simulink model "double_track_dynamics_model"  (R2023b)
settings: Solver=VariableStepAuto  StartTime=0.0  StopTime=10.0  RelTol=1e-3
undefined symbols (not defined in the file or in its folder): a, b, mass_total, track_width_front, track_width_rear, yaw_polar_inertia
settings Model: Creator=bglen  LastModifiedBy=bglen

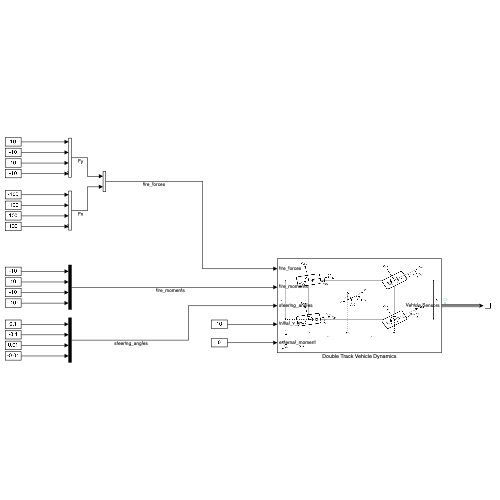
[thumbnail: Simulink's stored preview of the top-level diagram]
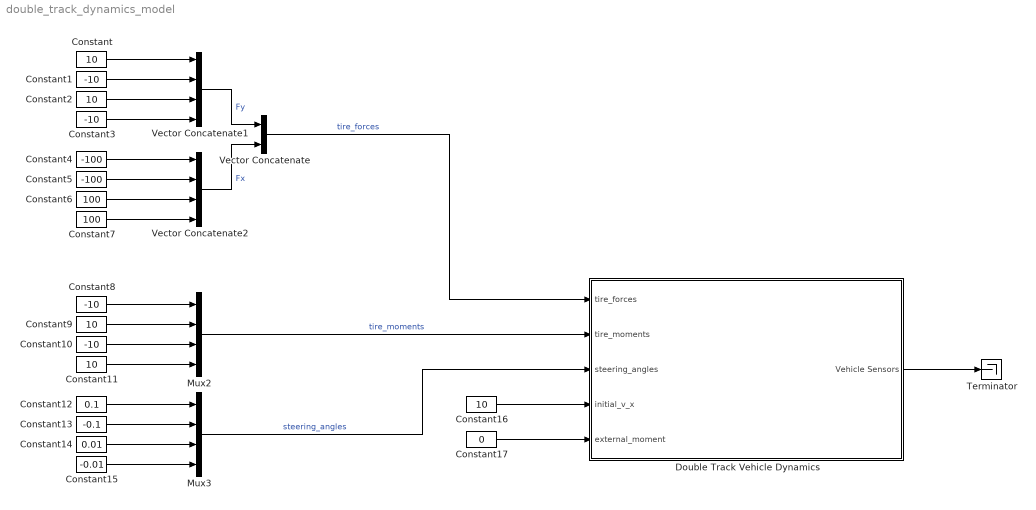
== system double_track_dynamics_model ==
  Constant{,2,9,11,16} (5 alike) : Constant  Value=10
  Constant{1,3,8,10} (4 alike) : Constant  Value=-10
  Constant12 : Constant  Value=0.1
  Constant13 : Constant  Value=-0.1
  Constant14 : Constant  Value=0.01
  Constant15 : Constant  Value=-0.01
  Constant17 : Constant  Value=0
  Constant4 : Constant  Value=-100
  Constant5 : Constant  Value=-100
  Constant6 : Constant  Value=100
  Constant7 : Constant  Value=100
  Double Track Vehicle Dynamics : Subsystem
      mask Display: image('double_track_diagram.png');
  Mux2 : Mux
  Mux3 : Mux
  Terminator : Terminator
  Vector Concatenate : Concatenate  Mode=Multidimensional array
  Vector Concatenate1 : Concatenate  NumInputs=4  Mode=Multidimensional array  ConcatenateDimension=2
  Vector Concatenate2 : Concatenate  NumInputs=4  Mode=Multidimensional array  ConcatenateDimension=2
  wires:
  Vector Concatenate/1 -> Double Track Vehicle Dynamics/1(tire_forces)  "tire_forces"
  Mux2/1 -> Double Track Vehicle Dynamics/2(tire_moments)  "tire_moments"
  Mux3/1 -> Double Track Vehicle Dynamics/3(steering_angles)  "steering_angles"
  Constant16/1 -> Double Track Vehicle Dynamics/4(initial_v_x)
  Double Track Vehicle Dynamics/1(Vehicle Sensors) -> Terminator/1
  Constant/1 -> Vector Concatenate1/1
  Constant2/1 -> Vector Concatenate1/3
  Constant3/1 -> Vector Concatenate1/4
  Constant6/1 -> Vector Concatenate2/3
  Constant7/1 -> Vector Concatenate2/4
  Constant4/1 -> Vector Concatenate2/1
  Constant5/1 -> Vector Concatenate2/2
  Vector Concatenate2/1 -> Vector Concatenate/2  "Fx"
  Constant9/1 -> Mux2/2
  Constant11/1 -> Mux2/4
  Constant8/1 -> Mux2/1
  Constant10/1 -> Mux2/3
  Constant13/1 -> Mux3/2
  Constant15/1 -> Mux3/4
  Constant12/1 -> Mux3/1
  Constant14/1 -> Mux3/3
  Constant1/1 -> Vector Concatenate1/2
  Vector Concatenate1/1 -> Vector Concatenate/1  "Fy"
  Constant17/1 -> Double Track Vehicle Dynamics/5(external_moment)

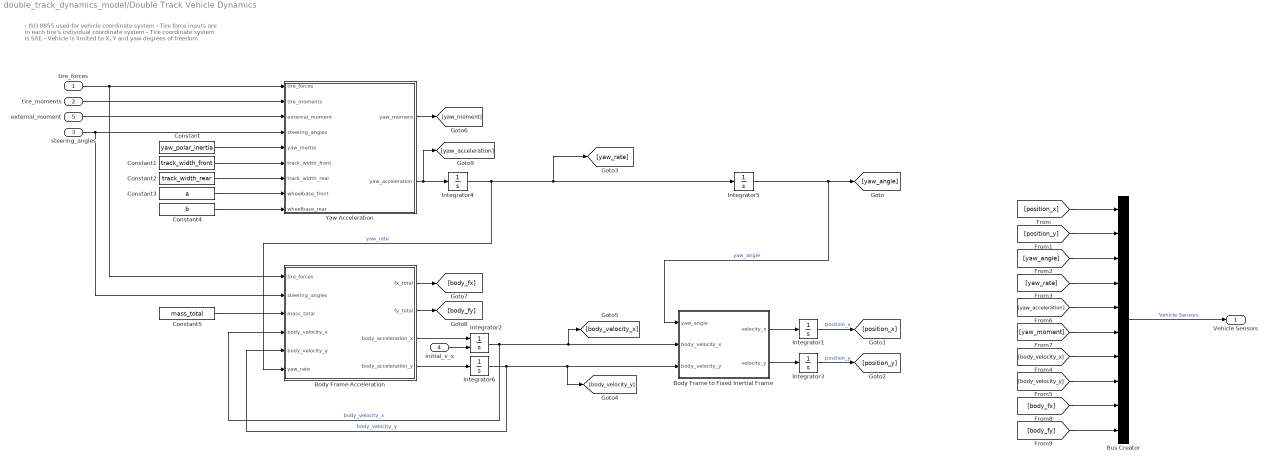
== system double_track_dynamics_model/Double Track Vehicle Dynamics ==
  note: - ISO 8855 used for vehicle coordinate system
      | - Tire force inputs are in each tire's individual coordinate system
      | - Tire coordinate system is SAE
      | - Vehicle is limited to X, Y and yaw degrees of freedom
  tire_forces : Inport
  tire_moments : Inport  Port=2
  steering_angles : Inport  Port=3
  initial_v_x : Inport  Port=4
  external_moment : Inport  Port=5
  Body Frame Acceleration : MATLAB Function  TreatAsAtomicUnit=on
  Body Frame to Fixed Inertial Frame : MATLAB Function  TreatAsAtomicUnit=on
  Bus Creator : BusCreator  Inputs=10
  Constant : Constant  Value=yaw_polar_inertia
  Constant1 : Constant  Value=track_width_front
  Constant2 : Constant  Value=track_width_rear
  Constant3 : Constant  Value=a
  Constant4 : Constant  Value=b
  Constant5 : Constant  Value=mass_total
  Integrator{1,3..6} (5 alike) : Integrator
  Integrator2 : Integrator  InitialConditionSource=external
  Yaw Acceleration : MATLAB Function  TreatAsAtomicUnit=on
  Vehicle Sensors : Outport
  wires:
  tire_moments/1 -> Yaw Acceleration/2(tire_moments)
  Bus Creator/1 -> Vehicle Sensors/1  "Vehicle Sensors"
  [yaw_rate] -> Bus Creator/4
  [position_y] -> Bus Creator/2
  Body Frame Acceleration/4(body_acceleration_y) -> Integrator6/1
  [position_x] -> Bus Creator/1
  steering_angles/1 -> Yaw Acceleration/4(steering_angles), Body Frame Acceleration/2(steering_angles)
  Integrator2/1 -> Body Frame Acceleration/4(body_velocity_x), [body_velocity_x], Body Frame to Fixed Inertial Frame/2(body_velocity_x)  "body_velocity_x"
  Body Frame to Fixed Inertial Frame/2(velocity_y) -> Integrator3/1
  Integrator1/1 -> [position_x]  "position_x"
  initial_v_x/1 -> Integrator2/2
  Integrator5/1 -> [yaw_angle], Body Frame to Fixed Inertial Frame/1(yaw_angle)  "yaw_angle"
  Integrator3/1 -> [position_y]  "position_y"
  [yaw_angle] -> Bus Creator/3
  Body Frame to Fixed Inertial Frame/1(velocity_x) -> Integrator1/1
  tire_forces/1 -> Body Frame Acceleration/1(tire_forces), Yaw Acceleration/1(tire_forces)
  Integrator4/1 -> Body Frame Acceleration/6(yaw_rate), [yaw_rate], Integrator5/1  "yaw_rate"
  Integrator6/1 -> Body Frame Acceleration/5(body_velocity_y), [body_velocity_y], Body Frame to Fixed Inertial Frame/3(body_velocity_y)  "body_velocity_y"
  Constant/1 -> Yaw Acceleration/5(yaw_inertia)
  Constant4/1 -> Yaw Acceleration/9(wheelbase_rear)
  Constant3/1 -> Yaw Acceleration/8(wheelbase_front)
  Constant2/1 -> Yaw Acceleration/7(track_width_rear)
  Constant1/1 -> Yaw Acceleration/6(track_width_front)
  Yaw Acceleration/2(yaw_acceleration) -> [yaw_acceleration], Integrator4/1
  Body Frame Acceleration/3(body_acceleration_x) -> Integrator2/1
  Constant5/1 -> Body Frame Acceleration/3(mass_total)
  Yaw Acceleration/1(yaw_moment) -> [yaw_moment]
  Body Frame Acceleration/1(fx_total) -> [body_fx]
  Body Frame Acceleration/2(fy_total) -> [body_fy]
  [yaw_acceleration] -> Bus Creator/5
  [yaw_moment] -> Bus Creator/6
  [body_velocity_x] -> Bus Creator/7
  [body_velocity_y] -> Bus Creator/8
  [body_fx] -> Bus Creator/9
  [body_fy] -> Bus Creator/10
  external_moment/1 -> Yaw Acceleration/3(external_moment)

== matlab function double_track_dynamics_model/Double Track Vehicle Dynamics/Body Frame Acceleration ==
  data: tire_forces input; steering_angles input; fx_total output; fy_total output; body_acceleration_x output; body_acceleration_y output; mass_total input; body_velocity_x input; body_velocity_y input; yaw_rate input
%{

Solve the equation of motion for longitudianl acceleration

Sum(Fx) / mass = long_acceleration

%% Inputs:

Tire Forces [N]: tire_forces = [fy_fl, fy_fr, fy_rl, fy_rr; fx_fl, fx_fr, fx_rl, fx_rr]; 
Steering Angles [rad]: steering_angles = [delta_fl, delta_fr, delta_rl, delta_rr];

%% Outputs:

fx_total [N]
fy_total [N]
body_acceleration_x [m/s^2]
body_acceleration_y [m/s^2]

%}
function [fx_total, fy_total, body_acceleration_x, body_acceleration_y]  = fcn(tire_forces, steering_angles, mass_total, body_velocity_x, body_velocity_y, yaw_rate)

%% convert input matricies into individual forces for code clarity
fy_fl = tire_forces(1, 1);
fy_fr = tire_forces(1, 2);
fy_rl = tire_forces(1, 3);
fy_rr = tire_forces(1, 4);

fx_fl = tire_forces(2, 1);
fx_fr = tire_forces(2, 2);
fx_rl = tire_forces(2, 3);
fx_rr = tire_forces(2, 4);

delta_fl = steering_angles(1);
delta_fr = steering_angles(2);
delta_rl = steering_angles(3);
delta_rr = steering_angles(4);

%% Convert tire forces into vehicle body frame
fx_body_fl = fy_fl * sin(delta_fl) + fx_fl * cos(delta_fl);
fy_body_fl = fy_fl * cos(delta_fl) + fx_fl * sin(delta_fl);

fx_body_fr = fy_fr * sin(delta_fr) + fx_fr * cos(delta_fr);
fy_body_fr = fy_fr * cos(delta_fr) + fx_fr * sin(delta_fr);

fx_body_rl = fy_rl * sin(delta_rl) + fx_rl * cos(delta_rl);
fy_body_rl = fy_rl * cos(delta_rl) + fx_rl * sin(delta_rl);

fx_body_rr = fy_rr * sin(delta_rr) + fx_rr * cos(delta_rr);
fy_body_rr = fy_rr * cos(delta_rr) + fx_rr * sin(delta_rr);

%% Calculate Longitudinal force and acceleration
fx_total = fx_body_fl + fx_body_fr + fx_body_rl + fx_body_rr;
body_acceleration_x = (fx_total / mass_total) - (yaw_rate * body_velocity_y); % must account for the apparent coriolis force

%% Calculate Lateral force and acceleration
fy_total = (fy_body_fl + fy_body_fr + fy_body_rl + fy_body_rr) + (yaw_rate * body_velocity_x); % must account for the apparent coriolis force
body_acceleration_y = fy_total / mass_total;

== matlab function double_track_dynamics_model/Double Track Vehicle Dynamics/Body Frame to Fixed Inertial Frame ==
  data: yaw_angle input; velocity_x output; body_velocity_x input; body_velocity_y input; velocity_y output
%{
%% Double Track Vehicle Dynamics

%% Overview
These equations describe the vehicle dynamics of a double track vehicle
model for longitudinal & lateral directions, and in the yaw axis. The model
keeps track of a fixed inertial frame for vehicle position and orientation.
The vehicle forces and velocities are described in a body-fixed refernce
frame.

%}
function [velocity_x, velocity_y] = fcn(yaw_angle, body_velocity_x, body_velocity_y)

velocity_x = body_velocity_x * cos(yaw_angle) - body_velocity_y * sin(yaw_angle);
velocity_y = body_velocity_x * sin(yaw_angle) + body_velocity_y * cos(yaw_angle);

== matlab function double_track_dynamics_model/Double Track Vehicle Dynamics/Yaw Acceleration ==
  data: tire_forces input; yaw_moment output; tire_moments input; external_moment input; steering_angles input; yaw_inertia input; track_width_front input; track_width_rear input; wheelbase_front input; wheelbase_rear input; yaw_acceleration output
%{

Solve the equation of motion for acceleration around the yaw axis

Sum(M) / Izz = yaw_acceleration

%% Inputs:

Tire Forces [N]: tire_forces = [fy_fl, fy_fr, fy_rl, fy_rr; fx_fl, fx_fr, fx_rl, fx_rr]; 
Tire Moments [Nm]: tire_moments = [mz_fl, mz_fr, mz_rl, mz_rr];
external_moment [Nm]: external moment applied to vehicle CG position
Steering Angles [rad]: steering_angles = [delta_fl, delta_fr, delta_rl, delta_rr];

%% Outputs:

yaw_moment [Nm]
yaw_acceleration [rad/s^2]

%}
function [yaw_moment, yaw_acceleration]  = fcn(tire_forces, tire_moments, external_moment, steering_angles, yaw_inertia, track_width_front, track_width_rear, wheelbase_front, wheelbase_rear)

%% convert input matricies into individual forces for code clarity
fy_fl = tire_forces(1, 1);
fy_fr = tire_forces(1, 2);
fy_rl = tire_forces(1, 3);
fy_rr = tire_forces(1, 4);

fx_fl = tire_forces(2, 1);
fx_fr = tire_forces(2, 2);
fx_rl = tire_forces(2, 3);
fx_rr = tire_forces(2, 4);

mz_fl = tire_moments(1);
mz_fr = tire_moments(2);
mz_rl = tire_moments(3);
mz_rr = tire_moments(4);

delta_fl = steering_angles(1);
delta_fr = steering_angles(2);
delta_rl = steering_angles(3);
delta_rr = steering_angles(4);


%% Convert tire forces into vehicle body frame
fx_body_fl = fy_fl * sin(delta_fl) + fx_fl * cos(delta_fl);
fy_body_fl = fy_fl * cos(delta_fl) + fx_fl * sin(delta_fl);

fx_body_fr = fy_fr * sin(delta_fr) + fx_fr * cos(delta_fr);
fy_body_fr = fy_fr * cos(delta_fr) + fx_fr * sin(delta_fr);

fx_body_rl = fy_rl * sin(delta_rl) + fx_rl * cos(delta_rl);
fy_body_rl = fy_rl * cos(delta_rl) + fx_rl * sin(delta_rl);

fx_body_rr = fy_rr * sin(delta_rr) + fx_rr * cos(delta_rr);
fy_body_rr = fy_rr * cos(delta_rr) + fx_rr * sin(delta_rr);

%% Calculate moment contributions
m_fl = -fx_body_fl * track_width_front / 2 + fy_body_fl * wheelbase_front;
m_fr = fx_body_fr * track_width_front / 2 + fy_body_fr * wheelbase_front;
m_rl = -fx_body_rl * track_width_rear / 2 - fy_body_rl * wheelbase_rear;
m_rr = fx_body_rr * track_width_rear / 2 - fy_body_rr * wheelbase_rear;

%% Calculate total yaw moment & acceleration
yaw_moment = (m_fl + m_fr + m_rl + m_rr) + (mz_fl + mz_fr + mz_rl + mz_rr) + external_moment; % sum moments from tire forces and self-aligning moments
yaw_acceleration = yaw_moment / yaw_inertia;
